simulink model "four"  (R2020b)
settings: Solver=FixedStepDiscrete  StartTime=0.0  StopTime=10.0  RelTol=1e-3
settings Model: Creator=USER  LastModifiedBy=USER

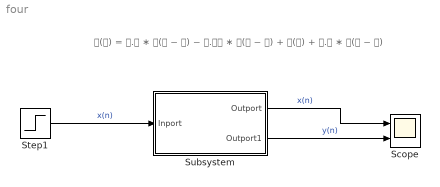
== system four ==
  note: 𝐲(𝐧) = 𝟎.𝟓 ∗ 𝐲(𝐧 − 𝟏) − 𝟎.𝟐𝟓 ∗ 𝐲(𝐧 − 𝟐) + 𝐱(𝐧) + 𝟎.𝟒 ∗ 𝐱(𝐧 − 𝟏)
  Scope : Scope  NumInputPorts=2
  Step1 : Step  SampleTime=0
  Subsystem : Subsystem
  wires:
  Step1/1 -> Subsystem/1(Inport)  "x(n)"
  Subsystem/1(Outport) -> Scope/1  "x(n)"
  Subsystem/2(Outport1) -> Scope/2  "y(n)"

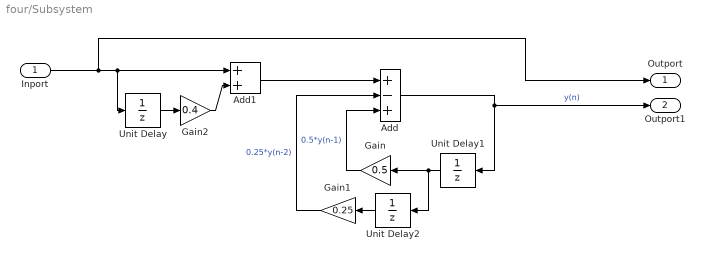
== system four/Subsystem ==
  Inport : Inport
  Add : Sum  Inputs=+-+
  Add1 : Sum
  Gain : Gain  Gain=0.5
  Gain1 : Gain  Gain=0.25
  Gain2 : Gain  Gain=0.4
  Unit Delay : UnitDelay  SampleTime=-1  HasFrameUpgradeWarning=on
  Unit Delay1 : UnitDelay  SampleTime=-1  HasFrameUpgradeWarning=on
  Unit Delay2 : UnitDelay  SampleTime=-1  HasFrameUpgradeWarning=on
  Outport : Outport
  Outport1 : Outport  Port=2
  wires:
  Inport/1 -> Outport/1, Unit Delay/1, Add1/1
  Add/1 -> Outport1/1, Unit Delay1/1  "y(n)"
  Add1/1 -> Add/1
  Gain1/1 -> Add/2  "0.25*y(n-2)"
  Unit Delay1/1 -> Unit Delay2/1, Gain/1
  Gain/1 -> Add/3  "0.5*y(n-1)"
  Unit Delay/1 -> Gain2/1
  Unit Delay2/1 -> Gain1/1
  Gain2/1 -> Add1/2
